simulink model "LSTMKerasTest"  (R2021a)
settings: Solver=VariableStepAuto  StartTime=0.0  StopTime=10  RelTol=1e-3
values from neighbouring files (symbols this model uses):
  delays = 99    [LSTMkeras_test.m]    (also in Net_Test.m = 31)
  x0 = zeros(length(sts_cnames),1)    [LSTMkeras_test.m]    (also in Net_Test.m)
  x0_f = cat(1,x0,zeros(3*4,1))    [LSTMkeras_test.m]    (also in Net_Test.m)
undefined symbols (not defined in the file or in its folder): norm_act, Ts
libraries: deeplib x1
settings Model: Creator=Eduardo  LastModifiedBy=Eduardo

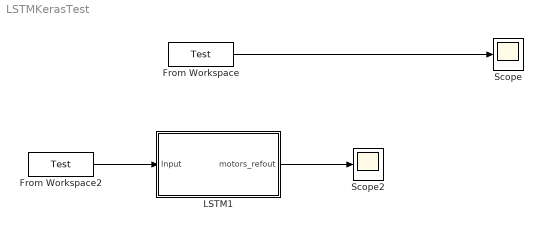
== system LSTMKerasTest ==
  From Workspace : FromWorkspace  VariableName=Test  SampleTime=5e-3
  From Workspace2 : FromWorkspace  VariableName=Test  SampleTime=5e-3
  LSTM1 : Subsystem  VariantControl=LSTM
  Scope : Scope
  Scope2 : Scope
  wires:
  From Workspace/1 -> Scope/1
  LSTM1/1(motors_refout) -> Scope2/1
  From Workspace2/1 -> LSTM1/1(Input)

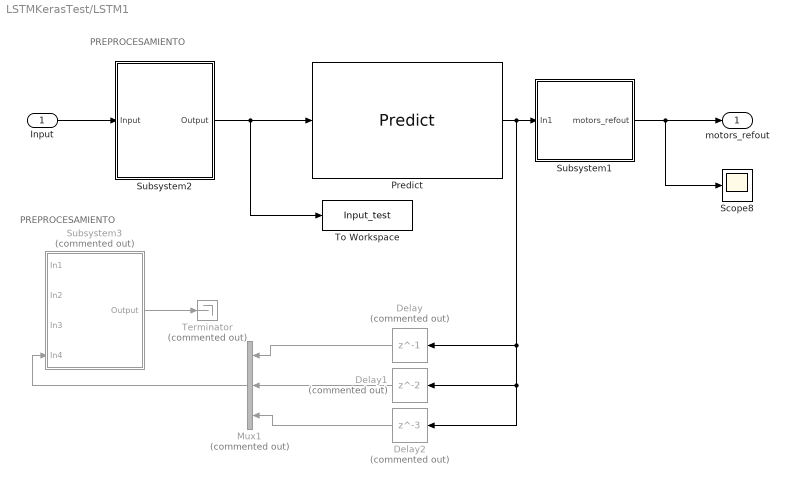
== system LSTMKerasTest/LSTM1 ==
  note: PREPROCESAMIENTO
  note: PREPROCESAMIENTO
  Input : Inport
  Delay : Delay  Commented=on  DelayLength=1
  Delay1 : Delay  Commented=on
  Delay2 : Delay  Commented=on  DelayLength=3
  Mux1 : Mux  Commented=on  Inputs=3
  Predict : deeplib/Predict  Network=Network from MATLAB function  NetworkFunction=myprediction  NetworkFilePath=mypre  MiniBatchSize=1024  InputDataFormats={ '', '' }  Predictions=on  Activations={}  ForceInterpretedSim=off  EnableDLNetwork=on
      settings: SourceProductBaseCode=NN
  Scope8 : Scope
  Subsystem1 : Subsystem
  Subsystem2 : Subsystem
  Subsystem3 : Subsystem  Commented=on
  Terminator : Terminator  Commented=on
  To Workspace : ToWorkspace  VariableName=Input_test  SaveFormat=Structure With Time  SampleTime=5e-3
      settings: Save2DSignal=2-D array (concatenate along first dimension)
  motors_refout : Outport
  wires:
  Subsystem3/1(Output) -> Terminator/1
  Subsystem2/1(Output) -> To Workspace/1, Predict/1
  Delay1/1 -> Mux1/2
  Subsystem1/1(motors_refout) -> motors_refout/1, Scope8/1
  Delay2/1 -> Mux1/3
  Delay/1 -> Mux1/1
  Predict/1 -> Delay/1, Delay2/1, Delay1/1, Subsystem1/1(In1)
  Mux1/1 -> Subsystem3/4(In4)
  Input/1 -> Subsystem2/1(Input)

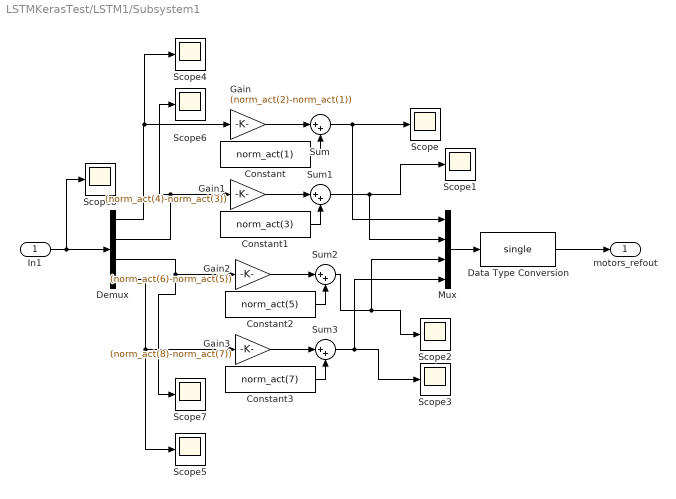
== system LSTMKerasTest/LSTM1/Subsystem1 ==
  In1 : Inport
  Constant : Constant  Value=norm_act(1)
  Constant1 : Constant  Value=norm_act(3)
  Constant2 : Constant  Value=norm_act(5)
  Constant3 : Constant  Value=norm_act(7)
  Data Type Conversion : DataTypeConversion  OutDataTypeStr=single
  Demux : Demux
  Gain : Gain  Gain=(norm_act(2)-norm_act(1))
  Gain1 : Gain  Gain=(norm_act(4)-norm_act(3))
  Gain2 : Gain  Gain=(norm_act(6)-norm_act(5))
  Gain3 : Gain  Gain=(norm_act(8)-norm_act(7))
  Mux : Mux
  Scope{,1..8} (9 alike) : Scope
  Sum{,1..3} (4 alike) : Sum  Inputs=|++
  motors_refout : Outport
  wires:
  In1/1 -> Scope8/1, Demux/1
  Demux/4 -> Scope5/1, Gain3/1
  Constant/1 -> Sum/2
  Gain/1 -> Sum/1
  Demux/1 -> Scope4/1, Gain/1
  Gain1/1 -> Sum1/1
  Constant1/1 -> Sum1/2
  Demux/2 -> Gain1/1, Scope6/1
  Gain2/1 -> Sum2/1
  Constant2/1 -> Sum2/2
  Demux/3 -> Scope7/1, Gain2/1
  Gain3/1 -> Sum3/1
  Constant3/1 -> Sum3/2
  Mux/1 -> Data Type Conversion/1
  Data Type Conversion/1 -> motors_refout/1
  Sum3/1 -> Mux/4, Scope3/1
  Sum1/1 -> Mux/2, Scope1/1
  Sum2/1 -> Mux/3, Scope2/1
  Sum/1 -> Mux/1, Scope/1

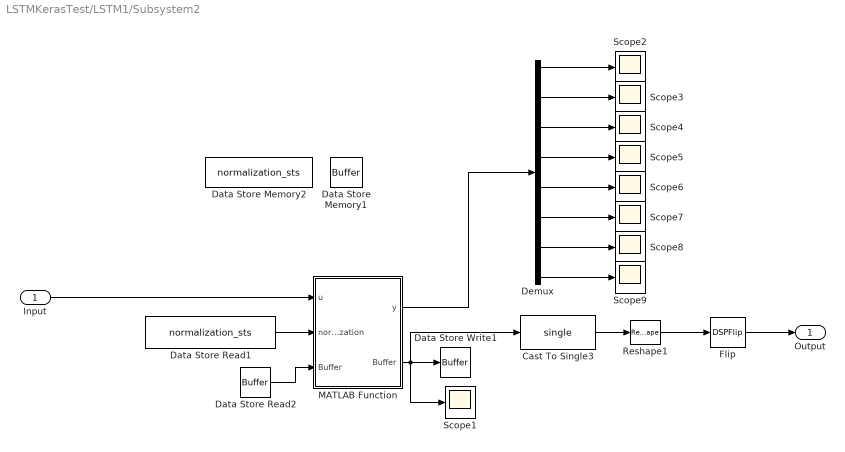
== system LSTMKerasTest/LSTM1/Subsystem2 ==
  Input : Inport
  Cast To Single3 : DataTypeConversion  OutDataTypeStr=single
  Data Store Memory1 : DataStoreMemory  DataStoreName=Buffer  ReadBeforeWriteMsg=warning  WriteAfterWriteMsg=warning  WriteAfterReadMsg=warning  InitialValue=repmat(x0,1,delays+1)  ShowAdditionalParam=off
  Data Store Memory2 : DataStoreMemory  DataStoreName=normalization_sts  ReadBeforeWriteMsg=warning  WriteAfterWriteMsg=warning  WriteAfterReadMsg=warning  InitialValue=normalization_sts  ShowAdditionalParam=off
  Data Store Read1 : DataStoreRead  DataStoreName=normalization_sts  IndexOptions=Index vector (dialog)  Indices=1  OutputSizes=1
  Data Store Read2 : DataStoreRead  DataStoreName=Buffer  IndexOptions=Index vector (dialog)  Indices=1  OutputSizes=1
  Data Store Write1 : DataStoreWrite  DataStoreName=Buffer  IndexOptions=Index vector (dialog)  Indices=1  OutputSizes=1
  Demux : Demux  Outputs=8
  Flip : DSPFlip  dim=Rows
  MATLAB Function : MATLAB Function  TreatAsAtomicUnit=on
  Reshape1 : Reshape  OutputDimensionality=Customize  OutputDimensions=[length(x0),delays+1]
  Scope{1..9} (9 alike) : Scope
  Output : Outport
  wires:
  Data Store Read1/1 -> MATLAB Function/2(normalization)
  Data Store Read2/1 -> MATLAB Function/3("Buffer ")
  MATLAB Function/2(Buffer) -> Cast To Single3/1, Scope1/1, Data Store Write1/1
  Cast To Single3/1 -> Reshape1/1
  Demux/1 -> Scope2/1
  MATLAB Function/1(y) -> Demux/1
  Demux/2 -> Scope3/1
  Demux/3 -> Scope4/1
  Demux/4 -> Scope5/1
  Demux/5 -> Scope6/1
  Demux/6 -> Scope7/1
  Demux/7 -> Scope8/1
  Demux/8 -> Scope9/1
  Input/1 -> MATLAB Function/1(u)
  Reshape1/1 -> Flip/1
  Flip/1 -> Output/1

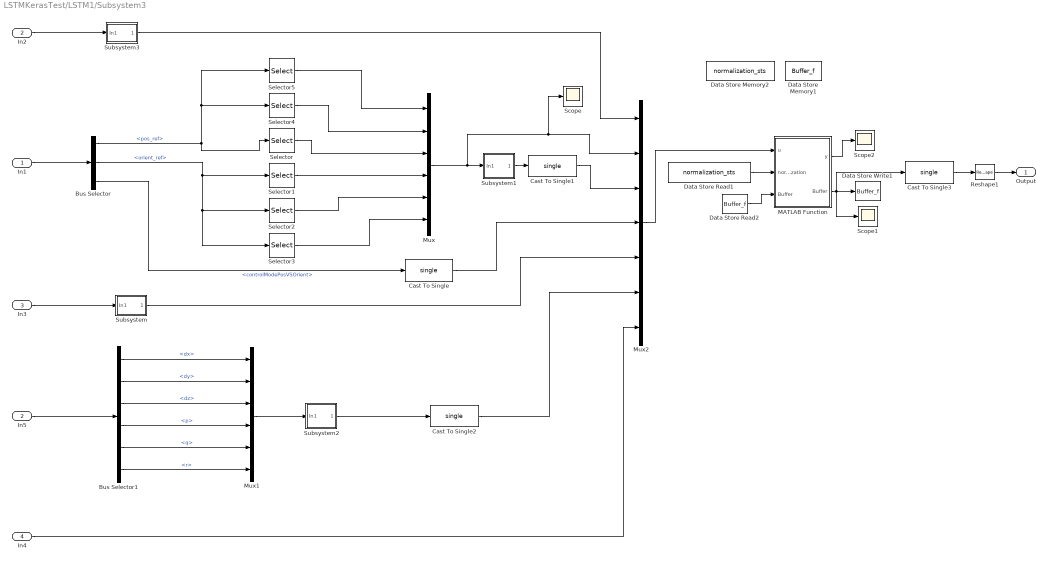
== system LSTMKerasTest/LSTM1/Subsystem3 ==
  In1 : Inport
  In2 : Inport  Port=2
  In3 : Inport  Port=3
  In4 : Inport  Port=4
  Bus Selector : BusSelector  OutputSignals=pos_ref,orient_ref,controlModePosVSOrient
  Bus Selector1 : BusSelector  OutputSignals=dx,dy,dz,p,q,r
  Cast To Single{,1..3} (4 alike) : DataTypeConversion  OutDataTypeStr=single
  Data Store Memory1 : DataStoreMemory  DataStoreName=Buffer_f  ReadBeforeWriteMsg=warning  WriteAfterWriteMsg=warning  WriteAfterReadMsg=warning  InitialValue=repmat(x0_f,1,delays+1)  ShowAdditionalParam=off
  Data Store Memory2 : DataStoreMemory  DataStoreName=normalization_sts  ReadBeforeWriteMsg=warning  WriteAfterWriteMsg=warning  WriteAfterReadMsg=warning  InitialValue=normalization_sts  ShowAdditionalParam=off
  Data Store Read1 : DataStoreRead  DataStoreName=normalization_sts  IndexOptions=Index vector (dialog)  Indices=1  OutputSizes=1
  Data Store Read2 : DataStoreRead  DataStoreName=Buffer_f  IndexOptions=Index vector (dialog)  Indices=1  OutputSizes=1
  Data Store Write1 : DataStoreWrite  DataStoreName=Buffer_f  IndexOptions=Index vector (dialog)  Indices=1  OutputSizes=1
  In5 : InportShadow  Port=2
  MATLAB Function : MATLAB Function  TreatAsAtomicUnit=on
  Mux : Mux  Inputs=6
  Mux1 : Mux  Inputs=6
  Mux2 : Mux  Inputs=7
      settings: DisplayOption=signals
  Reshape1 : Reshape  OutputDimensionality=Customize  OutputDimensions=[length(x0_f),delays+1]
  Scope : Scope
  Scope1 : Scope
  Scope2 : Scope
  Selector : Selector  InputPortWidth=3  IndexOptions=Index vector (dialog)  Indices=[3]  OutputSizes=1
  Selector1 : Selector  InputPortWidth=3  IndexOptions=Index vector (dialog)  Indices=[1]  OutputSizes=1
  Selector2 : Selector  InputPortWidth=3  IndexOptions=Index vector (dialog)  Indices=[3]  OutputSizes=1
  Selector3 : Selector  InputPortWidth=3  IndexOptions=Index vector (dialog)  Indices=[2]  OutputSizes=1
  Selector4 : Selector  InputPortWidth=3  IndexOptions=Index vector (dialog)  Indices=[2]  OutputSizes=1
  Selector5 : Selector  InputPortWidth=3  IndexOptions=Index vector (dialog)  Indices=[1]  OutputSizes=1
  Subsystem : Subsystem
  Subsystem1 : Subsystem
  Subsystem2 : Subsystem
  Subsystem3 : Subsystem
  Output : Outport
  wires:
  In1/1 -> Bus Selector/1
  Bus Selector/2 -> Selector3/1, Selector2/1, Selector1/1  "<orient_ref>"
  Bus Selector/1 -> Selector/1, Selector5/1, Selector4/1  "<pos_ref>"
  Selector5/1 -> Mux/1
  Selector4/1 -> Mux/2
  Selector/1 -> Mux/3
  Selector1/1 -> Mux/4
  Selector2/1 -> Mux/5
  Selector3/1 -> Mux/6
  Mux/1 -> Mux2/2, Scope/1, Subsystem1/1(In1)
  In5/1 -> Bus Selector1/1
  Bus Selector1/1 -> Mux1/1  "<dx>"
  Bus Selector1/2 -> Mux1/2  "<dy>"
  Bus Selector1/3 -> Mux1/3  "<dz>"
  Bus Selector1/4 -> Mux1/4  "<p>"
  Bus Selector1/5 -> Mux1/5  "<q>"
  Bus Selector1/6 -> Mux1/6  "<r>"
  Mux1/1 -> Subsystem2/1(In1)
  Mux2/1 -> MATLAB Function/1(u)
  MATLAB Function/1(y) -> Scope2/1
  In3/1 -> Subsystem/1(In1)
  In2/1 -> Subsystem3/1(In1)
  Bus Selector/3 -> Cast To Single/1  "<controlModePosVSOrient>"
  Cast To Single1/1 -> Mux2/3
  Subsystem1/1(Out1) -> Cast To Single1/1
  Subsystem2/1(Out1) -> Cast To Single2/1
  Data Store Read1/1 -> MATLAB Function/2(normalization)
  Data Store Read2/1 -> MATLAB Function/3("Buffer ")
  MATLAB Function/2(Buffer) -> Cast To Single3/1, Scope1/1, Data Store Write1/1
  Subsystem3/1(Out5) -> Mux2/1
  Cast To Single2/1 -> Mux2/6
  Subsystem/1(Out5) -> Mux2/5
  Cast To Single/1 -> Mux2/4
  In4/1 -> Mux2/7
  Cast To Single3/1 -> Reshape1/1
  Reshape1/1 -> Output/1

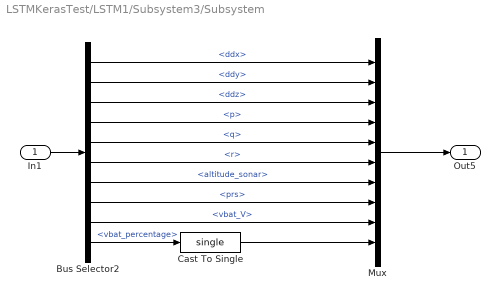
== system LSTMKerasTest/LSTM1/Subsystem3/Subsystem ==
  In1 : Inport
  Bus Selector2 : BusSelector  OutputSignals=ddx,ddy,ddz,p,q,r,altitude_sonar,prs,vbat_V,vbat_percentage
  Cast To Single : DataTypeConversion  OutDataTypeStr=single
  Mux : Mux  Inputs=10
  Out5 : Outport
  wires:
  In1/1 -> Bus Selector2/1
  Bus Selector2/1 -> Mux/1  "<ddx>"
  Bus Selector2/2 -> Mux/2  "<ddy>"
  Bus Selector2/3 -> Mux/3  "<ddz>"
  Bus Selector2/4 -> Mux/4  "<p>"
  Bus Selector2/5 -> Mux/5  "<q>"
  Bus Selector2/6 -> Mux/6  "<r>"
  Bus Selector2/7 -> Mux/7  "<altitude_sonar>"
  Bus Selector2/8 -> Mux/8  "<prs>"
  Bus Selector2/9 -> Mux/9  "<vbat_V>"
  Mux/1 -> Out5/1
  Bus Selector2/10 -> Cast To Single/1  "<vbat_percentage>"
  Cast To Single/1 -> Mux/10

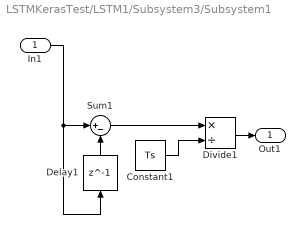
== system LSTMKerasTest/LSTM1/Subsystem3/Subsystem1 ==
  In1 : Inport
  Constant1 : Constant  Value=Ts
  Delay1 : Delay  DelayLength=1  InitialCondition=0
  Divide1 : Product  Inputs=*/
  Sum1 : Sum  Inputs=|+-
  Out1 : Outport
  wires:
  In1/1 -> Delay1/1, Sum1/1
  Constant1/1 -> Divide1/2
  Sum1/1 -> Divide1/1
  Delay1/1 -> Sum1/2
  Divide1/1 -> Out1/1

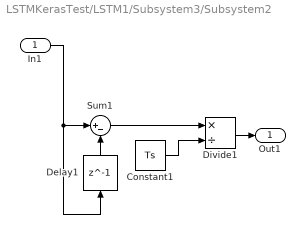
== system LSTMKerasTest/LSTM1/Subsystem3/Subsystem2 ==
  In1 : Inport
  Constant1 : Constant  Value=Ts
  Delay1 : Delay  DelayLength=1  InitialCondition=0
  Divide1 : Product  Inputs=*/
  Sum1 : Sum  Inputs=|+-
  Out1 : Outport
  wires:
  In1/1 -> Delay1/1, Sum1/1
  Constant1/1 -> Divide1/2
  Sum1/1 -> Divide1/1
  Delay1/1 -> Sum1/2
  Divide1/1 -> Out1/1

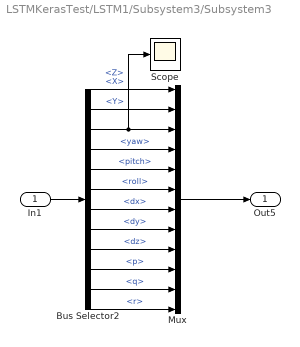
== system LSTMKerasTest/LSTM1/Subsystem3/Subsystem3 ==
  In1 : Inport
  Bus Selector2 : BusSelector  OutputSignals=X,Y,Z,yaw,pitch,roll,dx,dy,dz,p,q,r
  Mux : Mux  Inputs=12
  Scope : Scope
  Out5 : Outport
  wires:
  In1/1 -> Bus Selector2/1
  Mux/1 -> Out5/1
  Bus Selector2/1 -> Mux/1  "<X>"
  Bus Selector2/2 -> Mux/2  "<Y>"
  Bus Selector2/3 -> Scope/1, Mux/3  "<Z>"
  Bus Selector2/4 -> Mux/4  "<yaw>"
  Bus Selector2/5 -> Mux/5  "<pitch>"
  Bus Selector2/6 -> Mux/6  "<roll>"
  Bus Selector2/7 -> Mux/7  "<dx>"
  Bus Selector2/8 -> Mux/8  "<dy>"
  Bus Selector2/9 -> Mux/9  "<dz>"
  Bus Selector2/10 -> Mux/10  "<p>"
  Bus Selector2/11 -> Mux/11  "<q>"
  Bus Selector2/12 -> Mux/12  "<r>"

== matlab function LSTMKerasTest/LSTM1/Subsystem2/MATLAB Function ==
  data: u input; y output; normalization input; Buffer input; Buffer output
function [y,Buffer] = fcn(u, normalization, Buffer)

y=zeros(1,length(normalization(:,1)));

for i=1:length(normalization(:,1))
    %disp(normalization(:,3))
    if normalization(i,2)==normalization(i,1)
        y(1,i)=u(normalization(i,3));
    else
        y(1,i)=((u(normalization(i,3))-normalization(i,2))/(normalization(i,1)-normalization(i,2)));   
    end
    if y(1,i)>1 | y(1,i)<0
        disp("Fuera de los limites")
    end
    if y(1,i)==Inf
        disp("Infinito!!")
        disp(y(1,i))
    end
    if y(1,i)>1
        disp("Fuera de los limites")
    end
end

Buffer=circshift(Buffer,[0 1]);
sizeBuffer=(size(Buffer));
Buffer(:,1)=y;

== matlab function LSTMKerasTest/LSTM1/Subsystem3/MATLAB Function ==
  data: u input; y output; normalization input; Buffer input; Buffer output
function [y,Buffer] = fcn(u, normalization, Buffer)

y=zeros(1,length(normalization(:,1)));

for i=1:length(normalization(:,1))
    if normalization(i,2)==normalization(i,1)
        y(1,i)=u(normalization(i,3))
    else
        y(1,i)=((u(normalization(i,3))-normalization(i,2))/(normalization(i,1)-normalization(i,2)));   
    end
    if y(1,i)>1 | y(1,i)<0
        disp("Fuera de los limites")
    end
    if y(1,i)==Inf
        disp(y(1,i))
    end
end

Buffer=circshift(Buffer,[0 1]);
disp("OUT OF THE FEEDBACK")
disp(size(u(length(u)+1-(4*3):end)))
disp(size(y))
%Buffer=Buffer;
Buffer(:,1)=cat(2,y,u(length(u)+1-(4*3):end))
disp(size(Buffer(:,1)));
